simulink model "Resorte_No_Lineal"  (R2018a)
settings: Solver=VariableStepAuto  StartTime=0.0  StopTime=20  RelTol=1e-3
InitFcn:
  | m=10;
  | b=4;
  | k=5;
  | Kp=5*1;
  | Kv=2*sqrt(Kp);
libraries: roblocks x2
settings Model: Creator=Owner  LastModifiedBy=Federico

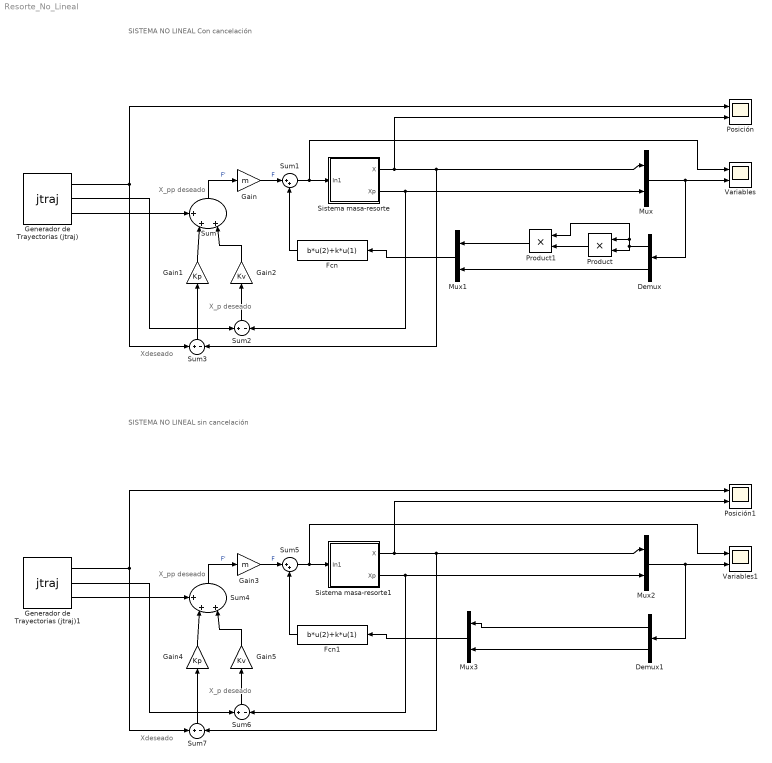
== system Resorte_No_Lineal ==
  note: SISTEMA NO LINEAL Con cancelación
  note: Xdeseado
  note: X_p
      | deseado
  note: X_pp
      | deseado
  note: Xdeseado
  note: X_p
      | deseado
  note: X_pp
      | deseado
  note: SISTEMA NO LINEAL sin cancelación
  Demux : Demux  Outputs=2
  Demux1 : Demux  Outputs=2
  Fcn : Fcn  Expr=b*u(2)+k*u(1)
  Fcn1 : Fcn  Expr=b*u(2)+k*u(1)
  Gain : Gain  Gain=m
  Gain1 : Gain  Gain=Kp
  Gain2 : Gain  Gain=Kv
  Gain3 : Gain  Gain=m
  Gain4 : Gain  Gain=Kp
  Gain5 : Gain  Gain=Kv
  Generador de Trayectorias (jtraj) : roblocks/Toolbox/jtraj  q0=[5 ]  qf=[-1]  tmax=10  ts=0.02
  Generador de Trayectorias (jtraj)1 : roblocks/Toolbox/jtraj  q0=[5 ]  qf=[-1]  tmax=10  ts=0.02
  Mux{,1..3} (4 alike) : Mux  Inputs=2
  Posición : Scope  NumInputPorts=2
  Posición1 : Scope  NumInputPorts=2
  Product : Product
  Product1 : Product
  Sistema masa-resorte : Subsystem
  Sistema masa-resorte1 : Subsystem
  Sum : Sum  Inputs=+++|
  Sum1 : Sum  Inputs=|++
  Sum{2..3,6..7} (4 alike) : Sum  Inputs=+-
  Sum4 : Sum  Inputs=+++|
  Sum5 : Sum  Inputs=|++
  Variables : Scope  NumInputPorts=2
  Variables1 : Scope  NumInputPorts=2
  wires:
  Fcn/1 -> Sum1/2
  Sum1/1 -> Variables/1, Sistema masa-resorte/1(In1)
  Sistema masa-resorte/1(X) -> Posición/2, Mux/1, Sum3/2
  Mux/1 -> Demux/1, Variables/2
  Sistema masa-resorte/2(Xp) -> Sum2/2, Mux/2
  Gain/1 -> Sum1/1  "F"
  Sum/1 -> Gain/1  "F'"
  Sum2/1 -> Gain2/1
  Generador de Trayectorias (jtraj)/2 -> Sum2/1
  Generador de Trayectorias (jtraj)/1 -> Posición/1, Sum3/1
  Sum3/1 -> Gain1/1
  Gain2/1 -> Sum/3
  Gain1/1 -> Sum/2
  Generador de Trayectorias (jtraj)/3 -> Sum/1
  Product/1 -> Product1/2
  Mux1/1 -> Fcn/1
  Product1/1 -> Mux1/1
  Demux/2 -> Mux1/2
  Demux/1 -> Product1/1, Product/1, Product/2
  Demux1/2 -> Mux3/2
  Sum5/1 -> Variables1/1, Sistema masa-resorte1/1(In1)
  Sum7/1 -> Gain4/1
  Mux3/1 -> Fcn1/1
  Gain5/1 -> Sum4/3
  Gain4/1 -> Sum4/2
  Sistema masa-resorte1/2(Xp) -> Sum6/2, Mux2/2
  Generador de Trayectorias (jtraj)1/1 -> Posición1/1, Sum7/1
  Generador de Trayectorias (jtraj)1/3 -> Sum4/1
  Generador de Trayectorias (jtraj)1/2 -> Sum6/1
  Demux1/1 -> Mux3/1
  Sum4/1 -> Gain3/1  "F'"
  Sum6/1 -> Gain5/1
  Fcn1/1 -> Sum5/2
  Mux2/1 -> Demux1/1, Variables1/2
  Sistema masa-resorte1/1(X) -> Posición1/2, Mux2/1, Sum7/2
  Gain3/1 -> Sum5/1  "F"

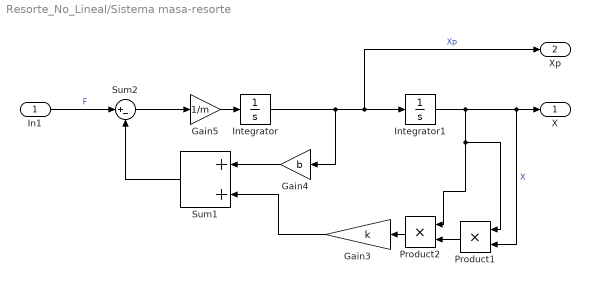
== system Resorte_No_Lineal/Sistema masa-resorte ==
  In1 : Inport
  Gain3 : Gain  Gain=k
  Gain4 : Gain  Gain=b
  Gain5 : Gain  Gain=1/m
  Integrator : Integrator
  Integrator1 : Integrator  InitialCondition=5
  Product1 : Product
  Product2 : Product
  Sum1 : Sum
  Sum2 : Sum  Inputs=|+-
  X : Outport
  Xp : Outport  Port=2
  wires:
  Sum1/1 -> Sum2/2
  Gain3/1 -> Sum1/2
  Gain5/1 -> Integrator/1
  Sum2/1 -> Gain5/1
  In1/1 -> Sum2/1  "F"
  Integrator1/1 -> Product1/1, Product2/1, Product1/2, X/1  "X"
  Gain4/1 -> Sum1/1
  Integrator/1 -> Integrator1/1, Xp/1, Gain4/1  "Xp"
  Product1/1 -> Product2/2
  Product2/1 -> Gain3/1

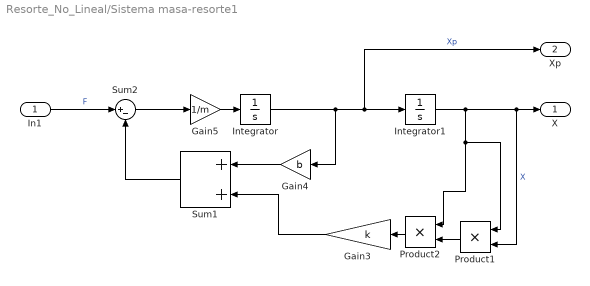
== system Resorte_No_Lineal/Sistema masa-resorte1 ==
  In1 : Inport
  Gain3 : Gain  Gain=k
  Gain4 : Gain  Gain=b
  Gain5 : Gain  Gain=1/m
  Integrator : Integrator
  Integrator1 : Integrator  InitialCondition=5
  Product1 : Product
  Product2 : Product
  Sum1 : Sum
  Sum2 : Sum  Inputs=|+-
  X : Outport
  Xp : Outport  Port=2
  wires:
  Sum1/1 -> Sum2/2
  Gain3/1 -> Sum1/2
  Gain5/1 -> Integrator/1
  Sum2/1 -> Gain5/1
  In1/1 -> Sum2/1  "F"
  Integrator1/1 -> Product1/1, Product2/1, Product1/2, X/1  "X"
  Gain4/1 -> Sum1/1
  Integrator/1 -> Integrator1/1, Xp/1, Gain4/1  "Xp"
  Product1/1 -> Product2/2
  Product2/1 -> Gain3/1
